simulink model "TrimControlSystemDesigner"  (R2026a)
settings: Solver=VariableStepAuto
undefined symbols (not defined in the file or in its folder): RCAM_Model_D
settings Model: Creator=nuris  LastModifiedBy=nuris

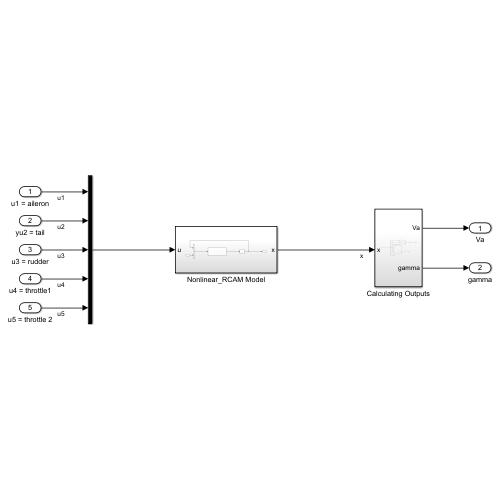
[thumbnail: Simulink's stored preview of the top-level diagram]
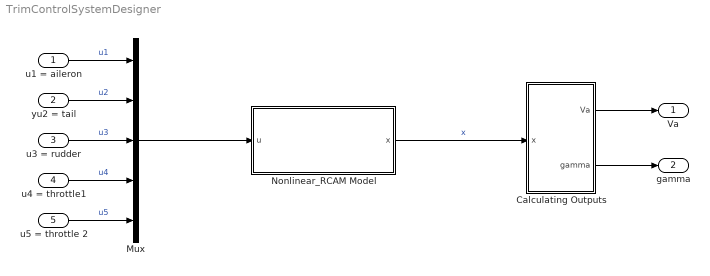
== system TrimControlSystemDesigner ==
  u1 = aileron : Inport
  yu2 = tail : Inport  Port=2
  u3 = rudder : Inport  Port=3
  u4 = throttle1 : Inport  Port=4
  u5 = throttle 2 : Inport  Port=5
  Calculating Outputs : Subsystem
  Mux : Mux  Inputs=5
  Nonlinear_RCAM Model : Subsystem
  Va : Outport
  gamma : Outport  Port=2
  wires:
  Mux/1 -> Nonlinear_RCAM Model/1(u)
  u1 = aileron/1 -> Mux/1  "u1"
  yu2 = tail/1 -> Mux/2  "u2"
  u3 = rudder/1 -> Mux/3  "u3"
  u4 = throttle1/1 -> Mux/4  "u4"
  u5 = throttle 2/1 -> Mux/5  "u5"
  Nonlinear_RCAM Model/1(x) -> Calculating Outputs/1(x)  "x"
  Calculating Outputs/1(Va) -> Va/1
  Calculating Outputs/2(gamma) -> gamma/1

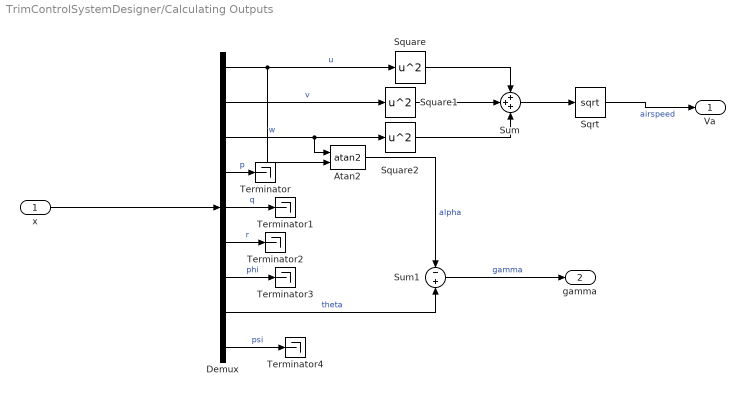
== system TrimControlSystemDesigner/Calculating Outputs ==
  x : Inport
  Atan2 : Trigonometry  Operator=atan2
  Demux : Demux  Outputs=9
  Sqrt : Sqrt
  Square : Math  Operator=square
  Square1 : Math  Operator=square
  Square2 : Math  Operator=square
  Sum : Sum  Inputs=+++
  Sum1 : Sum  Inputs=-|+
  Terminator{,1..4} (5 alike) : Terminator
  Va : Outport
  gamma : Outport  Port=2
  wires:
  Sum1/1 -> gamma/1  "gamma"
  Demux/1 -> Atan2/2, Square/1  "u"
  Square2/1 -> Sum/3
  Square1/1 -> Sum/2
  Demux/2 -> Square1/1  "v"
  Demux/4 -> Terminator/1  "p"
  Demux/3 -> Atan2/1, Square2/1  "w"
  Square/1 -> Sum/1
  Atan2/1 -> Sum1/1  "alpha"
  Sum/1 -> Sqrt/1
  Demux/8 -> Sum1/2  "theta"
  x/1 -> Demux/1
  Demux/5 -> Terminator1/1  "q"
  Demux/6 -> Terminator2/1  "r"
  Demux/7 -> Terminator3/1  "phi"
  Demux/9 -> Terminator4/1  "psi"
  Sqrt/1 -> Va/1  "airspeed"

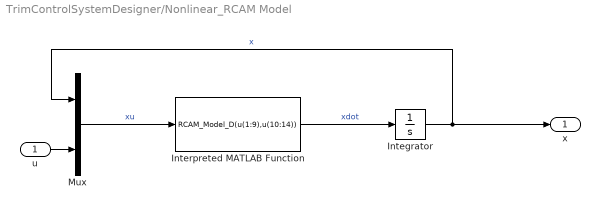
== system TrimControlSystemDesigner/Nonlinear_RCAM Model ==
  u : Inport
  Integrator : Integrator  InitialCondition=[85 ; 0 ; 0 ; 0; 0 ; 0 ; 0 ; 0; 0;]
  Interpreted MATLAB Function : MATLABFcn  MATLABFcn=RCAM_Model_D(u(1:9),u(10:14))
  Mux : Mux  Inputs=2
  x : Outport
  wires:
  u/1 -> Mux/2
  Mux/1 -> Interpreted MATLAB Function/1  "xu"
  Integrator/1 -> Mux/1, x/1  "x"
  Interpreted MATLAB Function/1 -> Integrator/1  "xdot"
